simulink model "es1_catena_aperta_1"  (R2014a)
settings: Solver=ode45  StartTime=0.0  StopTime=20.0  RelTol=1e-3
values from neighbouring files (symbols this model uses):
  beta = 0.02    [es1.m]
  Ka = 10    [es1.m]
  Km = 0.5    [es1.m]
  Ra = 1    [es1.m]
libraries: cstblocks x2
settings Model: Creator=HP  LastModifiedBy=HP
settings DataIOCC: InspectSignalLogs=on

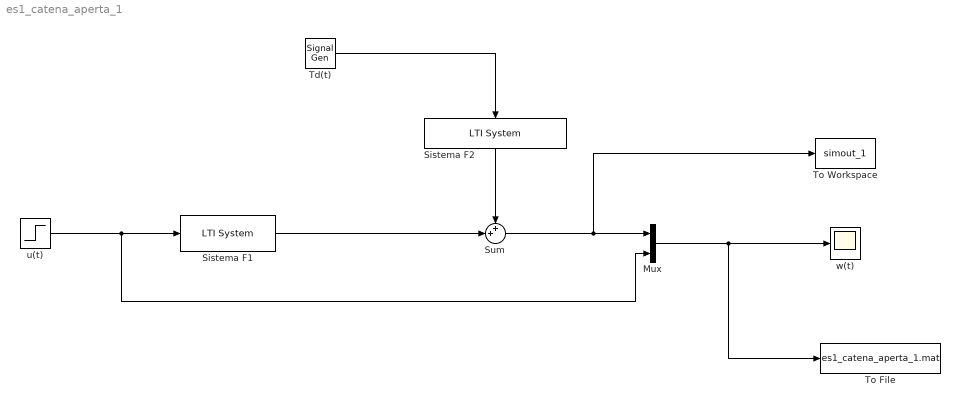
== system es1_catena_aperta_1 ==
  Mux : Mux  Inputs=2
  Sistema F1 : cstblocks/LTI System  sys=F1  IC=[]
  Sistema F2 : cstblocks/LTI System  sys=F2  IC=[]
  Sum : Sum  Inputs=++|
  Td(t) : SignalGenerator  WaveForm=square  Amplitude=0  Units=rad/sec
  To File : ToFile  Filename=es1_catena_aperta_1.mat  MatrixName=output_1  SaveFormat=Timeseries
  To Workspace : ToWorkspace  VariableName=simout_1  SaveFormat=Timeseries  SampleTime=-1
  u(t) : Step  Time=0  After=((Ka * Km) / (beta * Ra + Km*Km))^-1  SampleTime=0
  w(t) : Scope
  wires:
  u(t)/1 -> Mux/2, Sistema F1/1
  Sistema F2/1 -> Sum/1
  Sistema F1/1 -> Sum/2
  Sum/1 -> To Workspace/1, Mux/1
  Mux/1 -> To File/1, w(t)/1
  Td(t)/1 -> Sistema F2/1
